simulink model "SC_RHONN"  (R2024b)
settings: Solver=FixedStepAuto  StartTime=0.0  StopTime=inf  FixedStep=1e-5  RelTol=1e-3
model workspace (MAT data in the model file):
  test = 1
libraries: instrumentseriallib x2, simulink x2, spspowerguiLib x1
settings Model: SimulationMode=accelerator  Creator=Administrator  LastModifiedBy=l'c'c
settings RTWCC: GPUComputeCapability=3.5

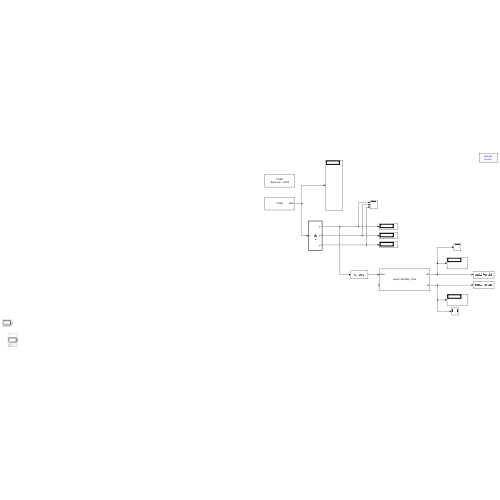
[thumbnail: Simulink's stored preview of the top-level diagram]
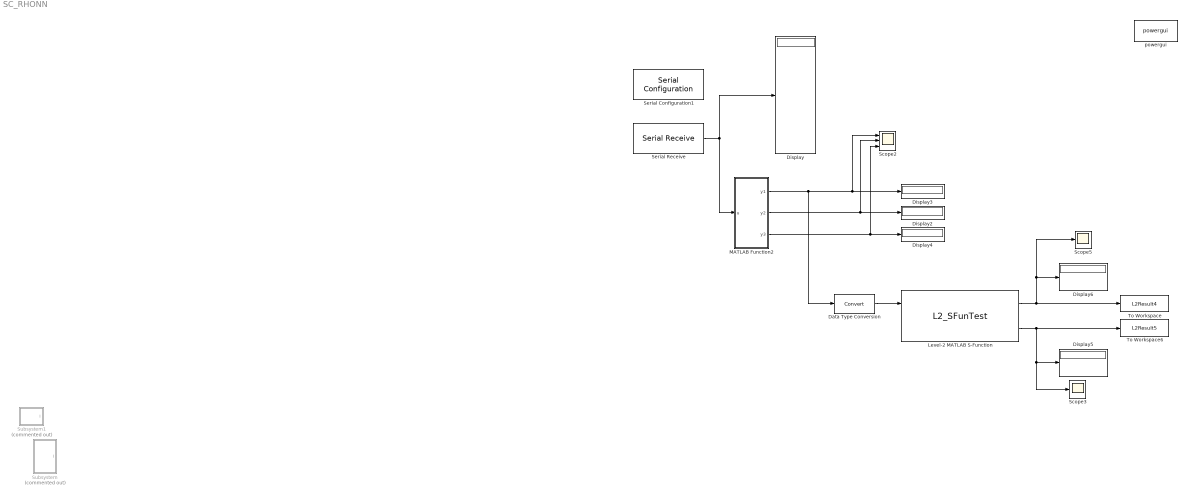
== system SC_RHONN ==
  Data Type Conversion : DataTypeConversion  SaturateOnIntegerOverflow=off  RndMeth=Floor
  Display{,2..6} (6 alike) : Display
      Display2 settings: Format=short_e
      Display3 settings: Format=short_e
      Display4 settings: Format=short_e
      Display5 settings: Priority=2
      Display6 settings: Priority=2
  Level-2 MATLAB S-Function : M-S-Function  Priority=1  FunctionName=L2_SFunTest  Parameters=Initial_Kp,Initial_Ki,Node_Num,Order_Num,Output_Num,kP_k,kQ,kR,cita  mask{Initial_Kp=0.75, Initial_Ki=20, Node_Num=2, Order_Num=3, Output_Num=2, kP_k=0.0001, kQ=0.001, kR=0.0011, cita=0.1}
      mask prompts: Initial_Kp "Initial Value of Kp"; Initial_Ki "Initial Value of Ki"; Node_Num "Node Number of RHONN"; Order_Num "Order Number of RHONN"; Output_Num "Output Number of RHONN"; kP_k "kP_k of RHONN"; kQ "kQ of RHONN"; kR "kR of RHONN"; cita "cita of RHONN"
      mask DialogControl ParameterGroupVar Prompt: 参数
      mask Display:
      | port_label('output', 1, 'Kp');
      | port_label('output', 2, 'Ki');
      | port_label('input', 1, 'Error');
      | 
      | disp('Level2_RHONN_CTRL');
  MATLAB Function2 : MATLAB Function  TreatAsAtomicUnit=on
  Scope2 : Scope  NumInputPorts=3
  Scope3 : Scope
  Scope5 : Scope
  Serial Configuration1 : instrumentseriallib/Serial Configuration  Priority=-200000  PortSel=COM5  Port=COM5  ComPort=COM5  BaudRate=19200  DataBits=8  Parity=none  StopBits=1  ByteOrder=little-endian  FlowControl=none  Timeout=1.0  SimulateUsing=Interpreted execution  BlockInModel=on  aMode=1
  Serial Receive : instrumentseriallib/Serial Receive  Priority=1  PortSel=COM5  Port=COM5  ComPort=COM5  DataType=int8  SaveDataType=uint8  ToggleHeader=off  Header=[]  ToggleDataSize=on  DataSize=[12 1]  ToggleTerminator=off  Terminator=<none>  CustomTerminator=[]  InputFormat=Column major  EnableBlockingMode=on  ActionDataUnavailable=Output last received value  ActionWhenDataUnavailable=Output last received value  CustomValue=0  SampleTime=-1  SimulateUsing=Interpreted execution  BlockInModel=on  aMode=1
  Subsystem : Subsystem  Commented=on
  Subsystem1 : Subsystem  Commented=on
  To Workspace : ToWorkspace  VariableName=L2Result4  SaveFormat=Timeseries  SampleTime=-1
  To Workspace6 : ToWorkspace  VariableName=L2Result5  SaveFormat=Timeseries  SampleTime=-1
  powergui : spspowerguiLib/powergui  Priority=1  SimulationMode=Discrete  SampleTime=1e-5  frequency=60  Iterations=50  frequencyindice=50  Pbase=100e6  ErrMax=1e-4  UnitsV=kV  UnitsW=MW  buscounter=0  FunctionMessages=off  echomessages=off  EnableUseOfTLC=off  CurrentSourceSwitches=off  DisableSnubberDevices=off  DisableRonSwitches=off  DisableVfSwitches=off  DisplayEquations=off  AutomaticDiscreteSolvers=off  SolverType=Tustin/Backward Euler (TBE)  Interpol=off  ExternalGateDelay=off  methode=off  Ts=100  x0status=blocks  SPID=on  SwTol=0  HookPort=off  NonlinearTolerance=1e-4  nMaxIteration=100  ContinueOnMaxIteration=off  RestoreLinks=warning  ResistiveCurrentMeasurement=off  Frange=[0:2:500]  Ylog=off  Xlog=on  ShowGrid=off  save=off  variable=ZData  structure=0  ZoomFFT=off  StartTime=0.0  cycles=1  DisplayStyle=1  fundamental=60  FreqAxis=off  MaxFrequency=1000  frequencyindicesteady=1  RmsSteady=1  display=off
  wires:
  Serial Receive/1 -> Display/1, MATLAB Function2/1(u)
  MATLAB Function2/3(y3) -> Scope2/3, Display4/1
  Level-2 MATLAB S-Function/1 -> Scope5/1, Display6/1, To Workspace/1
  Level-2 MATLAB S-Function/2 -> To Workspace6/1, Scope3/1, Display5/1
  Data Type Conversion/1 -> Level-2 MATLAB S-Function/1
  MATLAB Function2/1(y1) -> Scope2/1, Display3/1, Data Type Conversion/1
  MATLAB Function2/2(y2) -> Scope2/2, Display2/1

== system SC_RHONN/Subsystem ==
  Add2 : Sum  Inputs=++++
  Sine Wave3 : Sin  Amplitude=6  Frequency=2*pi*50  SampleTime=0
  Subsystem1 : Subsystem
  Subsystem6 : Subsystem
  Subsystem7 : Subsystem
  I : Outport
  wires:
  Subsystem6/1(Out1) -> Add2/4
  Subsystem1/1(Out1) -> Add2/3
  Add2/1 -> I/1
  Sine Wave3/1 -> Add2/1
  Subsystem7/1(Out1) -> Add2/2

== system SC_RHONN/Subsystem1 ==
  Add2 : Sum  Inputs=++++
  Constant : Constant  Value=400
  Subsystem1 : Subsystem
  Subsystem6 : Subsystem  Commented=on
  Subsystem7 : Subsystem
  I : Outport
  wires:
  Subsystem6/1(Out1) -> Add2/4
  Subsystem1/1(Out1) -> Add2/3
  Add2/1 -> I/1
  Constant/1 -> Add2/1
  Subsystem7/1(Out1) -> Add2/2

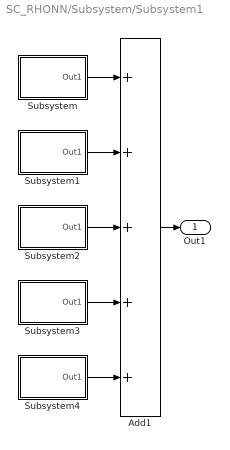
== system SC_RHONN/Subsystem/Subsystem1 ==
  Add1 : Sum  Inputs=+++++
  Subsystem : Subsystem
  Subsystem1 : Subsystem
  Subsystem2 : Subsystem
  Subsystem3 : Subsystem
  Subsystem4 : Subsystem
  Out1 : Outport
  wires:
  Subsystem1/1(Out1) -> Add1/2
  Subsystem3/1(Out1) -> Add1/4
  Subsystem4/1(Out1) -> Add1/5
  Subsystem2/1(Out1) -> Add1/3
  Subsystem/1(Out1) -> Add1/1
  Add1/1 -> Out1/1

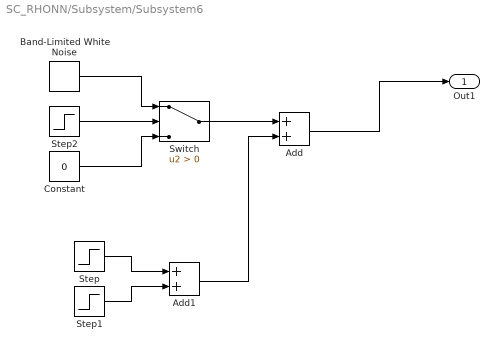
== system SC_RHONN/Subsystem/Subsystem6 ==
  Add : Sum
  Add1 : Sum
  Band-Limited White Noise : simulink/Sources/Band-Limited White Noise  Cov=[1e-5]  Ts=1e-3  seed=[23341]
  Constant : Constant  Value=0
  Step : Step  Time=0.024  After=0.3  SampleTime=0
  Step1 : Step  Time=0.026  After=-0.3  SampleTime=0
  Step2 : Step  Time=0.02  Before=1  After=0  SampleTime=0
  Switch : Switch  Criteria=u2 > Threshold  SaturateOnIntegerOverflow=off  InputSameDT=off
  Out1 : Outport
  wires:
  Add/1 -> Out1/1
  Step/1 -> Add1/1
  Constant/1 -> Switch/3
  Step1/1 -> Add1/2
  Step2/1 -> Switch/2
  Band-Limited White Noise/1 -> Switch/1
  Switch/1 -> Add/1
  Add1/1 -> Add/2

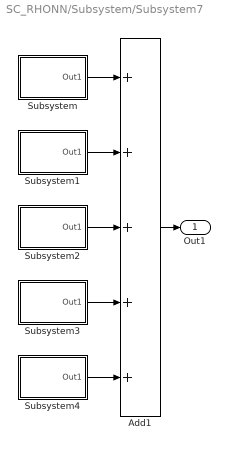
== system SC_RHONN/Subsystem/Subsystem7 ==
  Add1 : Sum  Inputs=+++++
  Subsystem : Subsystem
  Subsystem1 : Subsystem
  Subsystem2 : Subsystem
  Subsystem3 : Subsystem
  Subsystem4 : Subsystem
  Out1 : Outport
  wires:
  Add1/1 -> Out1/1
  Subsystem/1(Out1) -> Add1/1
  Subsystem2/1(Out1) -> Add1/3
  Subsystem4/1(Out1) -> Add1/5
  Subsystem3/1(Out1) -> Add1/4
  Subsystem1/1(Out1) -> Add1/2

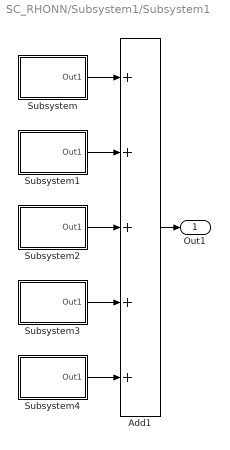
== system SC_RHONN/Subsystem1/Subsystem1 ==
  Add1 : Sum  Inputs=+++++
  Subsystem : Subsystem
  Subsystem1 : Subsystem
  Subsystem2 : Subsystem
  Subsystem3 : Subsystem
  Subsystem4 : Subsystem
  Out1 : Outport
  wires:
  Subsystem1/1(Out1) -> Add1/2
  Subsystem3/1(Out1) -> Add1/4
  Subsystem4/1(Out1) -> Add1/5
  Subsystem2/1(Out1) -> Add1/3
  Subsystem/1(Out1) -> Add1/1
  Add1/1 -> Out1/1

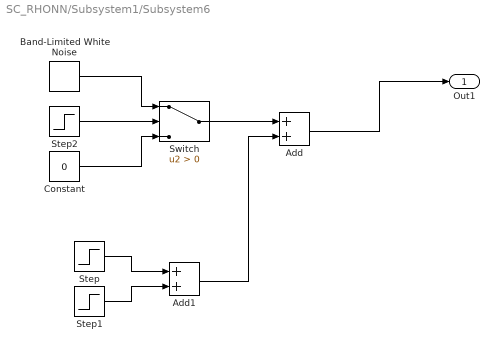
== system SC_RHONN/Subsystem1/Subsystem6 ==
  Add : Sum
  Add1 : Sum
  Band-Limited White Noise : simulink/Sources/Band-Limited White Noise  Cov=[1e-6]  Ts=0.0001  seed=[23341]
  Constant : Constant  Value=0
  Step : Step  Time=0.024  After=0.3  SampleTime=0
  Step1 : Step  Time=0.026  After=-0.3  SampleTime=0
  Step2 : Step  Time=0.02  Before=1  After=0  SampleTime=0
  Switch : Switch  Criteria=u2 > Threshold  SaturateOnIntegerOverflow=off  InputSameDT=off
  Out1 : Outport
  wires:
  Add/1 -> Out1/1
  Step/1 -> Add1/1
  Constant/1 -> Switch/3
  Step1/1 -> Add1/2
  Step2/1 -> Switch/2
  Band-Limited White Noise/1 -> Switch/1
  Switch/1 -> Add/1
  Add1/1 -> Add/2

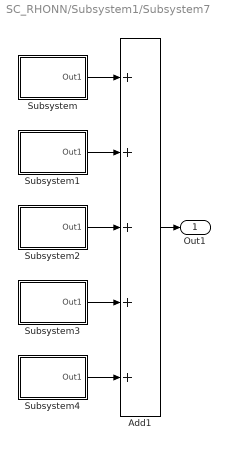
== system SC_RHONN/Subsystem1/Subsystem7 ==
  Add1 : Sum  Inputs=+++++
  Subsystem : Subsystem
  Subsystem1 : Subsystem
  Subsystem2 : Subsystem
  Subsystem3 : Subsystem
  Subsystem4 : Subsystem
  Out1 : Outport
  wires:
  Add1/1 -> Out1/1
  Subsystem/1(Out1) -> Add1/1
  Subsystem2/1(Out1) -> Add1/3
  Subsystem4/1(Out1) -> Add1/5
  Subsystem3/1(Out1) -> Add1/4
  Subsystem1/1(Out1) -> Add1/2

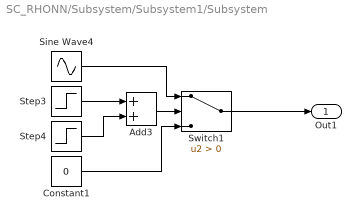
== system SC_RHONN/Subsystem/Subsystem1/Subsystem ==
  Add3 : Sum
  Constant1 : Constant  Value=0
  Sine Wave4 : Sin  Amplitude=6  Frequency=2*pi*50  Phase=pi  SampleTime=0
  Step3 : Step  Time=0.6  SampleTime=0
  Step4 : Step  Time=0.62  After=-1  SampleTime=0
  Switch1 : Switch  Criteria=u2 > Threshold  SaturateOnIntegerOverflow=off  InputSameDT=off
  Out1 : Outport
  wires:
  Switch1/1 -> Out1/1
  Step3/1 -> Add3/1
  Step4/1 -> Add3/2
  Add3/1 -> Switch1/2
  Sine Wave4/1 -> Switch1/1
  Constant1/1 -> Switch1/3

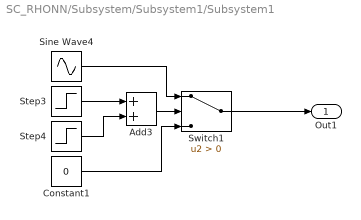
== system SC_RHONN/Subsystem/Subsystem1/Subsystem1 ==
  Add3 : Sum
  Constant1 : Constant  Value=0
  Sine Wave4 : Sin  Amplitude=5  Frequency=2*pi*50  Phase=pi  SampleTime=0
  Step3 : Step  Time=0.62  SampleTime=0
  Step4 : Step  Time=0.64  After=-1  SampleTime=0
  Switch1 : Switch  Criteria=u2 > Threshold  SaturateOnIntegerOverflow=off  InputSameDT=off
  Out1 : Outport
  wires:
  Constant1/1 -> Switch1/3
  Sine Wave4/1 -> Switch1/1
  Add3/1 -> Switch1/2
  Step4/1 -> Add3/2
  Step3/1 -> Add3/1
  Switch1/1 -> Out1/1

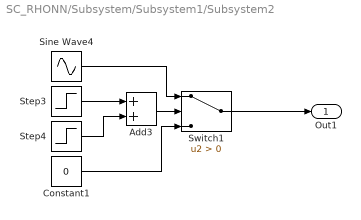
== system SC_RHONN/Subsystem/Subsystem1/Subsystem2 ==
  Add3 : Sum
  Constant1 : Constant  Value=0
  Sine Wave4 : Sin  Amplitude=4  Frequency=2*pi*50  Phase=pi  SampleTime=0
  Step3 : Step  Time=0.64  SampleTime=0
  Step4 : Step  Time=0.66  After=-1  SampleTime=0
  Switch1 : Switch  Criteria=u2 > Threshold  SaturateOnIntegerOverflow=off  InputSameDT=off
  Out1 : Outport
  wires:
  Switch1/1 -> Out1/1
  Step3/1 -> Add3/1
  Step4/1 -> Add3/2
  Add3/1 -> Switch1/2
  Sine Wave4/1 -> Switch1/1
  Constant1/1 -> Switch1/3

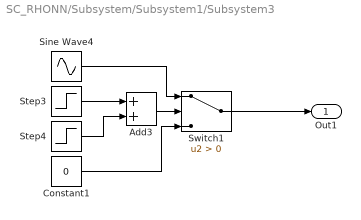
== system SC_RHONN/Subsystem/Subsystem1/Subsystem3 ==
  Add3 : Sum
  Constant1 : Constant  Value=0
  Sine Wave4 : Sin  Amplitude=3  Frequency=2*pi*50  Phase=pi  SampleTime=0
  Step3 : Step  Time=0.66  SampleTime=0
  Step4 : Step  Time=0.68  After=-1  SampleTime=0
  Switch1 : Switch  Criteria=u2 > Threshold  SaturateOnIntegerOverflow=off  InputSameDT=off
  Out1 : Outport
  wires:
  Constant1/1 -> Switch1/3
  Sine Wave4/1 -> Switch1/1
  Add3/1 -> Switch1/2
  Step4/1 -> Add3/2
  Step3/1 -> Add3/1
  Switch1/1 -> Out1/1

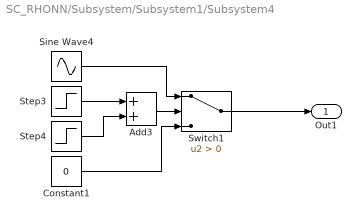
== system SC_RHONN/Subsystem/Subsystem1/Subsystem4 ==
  Add3 : Sum
  Constant1 : Constant  Value=0
  Sine Wave4 : Sin  Amplitude=2  Frequency=2*pi*50  Phase=pi  SampleTime=0
  Step3 : Step  Time=0.68  SampleTime=0
  Step4 : Step  Time=0.7  After=-1  SampleTime=0
  Switch1 : Switch  Criteria=u2 > Threshold  SaturateOnIntegerOverflow=off  InputSameDT=off
  Out1 : Outport
  wires:
  Switch1/1 -> Out1/1
  Step3/1 -> Add3/1
  Step4/1 -> Add3/2
  Add3/1 -> Switch1/2
  Sine Wave4/1 -> Switch1/1
  Constant1/1 -> Switch1/3

== system SC_RHONN/Subsystem/Subsystem7/Subsystem ==
  Add3 : Sum
  Constant1 : Constant  Value=0
  Sine Wave4 : Sin  Amplitude=6  Frequency=2*pi*50  Phase=2*pi  SampleTime=0
  Step3 : Step  Time=0.2  SampleTime=0
  Step4 : Step  Time=0.22  After=-1  SampleTime=0
  Switch1 : Switch  Criteria=u2 > Threshold  SaturateOnIntegerOverflow=off  InputSameDT=off
  Out1 : Outport
  wires:
  Constant1/1 -> Switch1/3
  Sine Wave4/1 -> Switch1/1
  Add3/1 -> Switch1/2
  Step4/1 -> Add3/2
  Step3/1 -> Add3/1
  Switch1/1 -> Out1/1

== system SC_RHONN/Subsystem/Subsystem7/Subsystem1 ==
  Add3 : Sum
  Constant1 : Constant  Value=0
  Sine Wave4 : Sin  Amplitude=5  Frequency=2*pi*50  Phase=2*pi  SampleTime=0
  Step3 : Step  Time=0.22  SampleTime=0
  Step4 : Step  Time=0.24  After=-1  SampleTime=0
  Switch1 : Switch  Criteria=u2 > Threshold  SaturateOnIntegerOverflow=off  InputSameDT=off
  Out1 : Outport
  wires:
  Switch1/1 -> Out1/1
  Step3/1 -> Add3/1
  Step4/1 -> Add3/2
  Add3/1 -> Switch1/2
  Sine Wave4/1 -> Switch1/1
  Constant1/1 -> Switch1/3

== system SC_RHONN/Subsystem/Subsystem7/Subsystem2 ==
  Add3 : Sum
  Constant1 : Constant  Value=0
  Sine Wave4 : Sin  Amplitude=4  Frequency=2*pi*50  Phase=2*pi  SampleTime=0
  Step3 : Step  Time=0.24  SampleTime=0
  Step4 : Step  Time=0.26  After=-1  SampleTime=0
  Switch1 : Switch  Criteria=u2 > Threshold  SaturateOnIntegerOverflow=off  InputSameDT=off
  Out1 : Outport
  wires:
  Constant1/1 -> Switch1/3
  Sine Wave4/1 -> Switch1/1
  Add3/1 -> Switch1/2
  Step4/1 -> Add3/2
  Step3/1 -> Add3/1
  Switch1/1 -> Out1/1

== system SC_RHONN/Subsystem/Subsystem7/Subsystem3 ==
  Add3 : Sum
  Constant1 : Constant  Value=0
  Sine Wave4 : Sin  Amplitude=3  Frequency=2*pi*50  Phase=2*pi  SampleTime=0
  Step3 : Step  Time=0.26  SampleTime=0
  Step4 : Step  Time=0.28  After=-1  SampleTime=0
  Switch1 : Switch  Criteria=u2 > Threshold  SaturateOnIntegerOverflow=off  InputSameDT=off
  Out1 : Outport
  wires:
  Switch1/1 -> Out1/1
  Step3/1 -> Add3/1
  Step4/1 -> Add3/2
  Add3/1 -> Switch1/2
  Sine Wave4/1 -> Switch1/1
  Constant1/1 -> Switch1/3

== system SC_RHONN/Subsystem/Subsystem7/Subsystem4 ==
  Add3 : Sum
  Constant1 : Constant  Value=0
  Sine Wave4 : Sin  Amplitude=2  Frequency=2*pi*50  Phase=2*pi  SampleTime=0
  Step3 : Step  Time=0.28  SampleTime=0
  Step4 : Step  Time=0.3  After=-1  SampleTime=0
  Switch1 : Switch  Criteria=u2 > Threshold  SaturateOnIntegerOverflow=off  InputSameDT=off
  Out1 : Outport
  wires:
  Constant1/1 -> Switch1/3
  Sine Wave4/1 -> Switch1/1
  Add3/1 -> Switch1/2
  Step4/1 -> Add3/2
  Step3/1 -> Add3/1
  Switch1/1 -> Out1/1

== system SC_RHONN/Subsystem1/Subsystem1/Subsystem ==
  Add3 : Sum
  Constant1 : Constant  Value=0
  Constant2 : Constant  Value=-10
  Step3 : Step  Time=0.6  SampleTime=0
  Step4 : Step  Time=0.62  After=-1  SampleTime=0
  Switch1 : Switch  Criteria=u2 > Threshold  SaturateOnIntegerOverflow=off  InputSameDT=off
  Out1 : Outport
  wires:
  Switch1/1 -> Out1/1
  Step3/1 -> Add3/1
  Step4/1 -> Add3/2
  Add3/1 -> Switch1/2
  Constant2/1 -> Switch1/1
  Constant1/1 -> Switch1/3

== system SC_RHONN/Subsystem1/Subsystem1/Subsystem1 ==
  Add3 : Sum
  Constant1 : Constant  Value=0
  Constant2 : Constant  Value=-8
  Step3 : Step  Time=0.62  SampleTime=0
  Step4 : Step  Time=0.64  After=-1  SampleTime=0
  Switch1 : Switch  Criteria=u2 > Threshold  SaturateOnIntegerOverflow=off  InputSameDT=off
  Out1 : Outport
  wires:
  Constant1/1 -> Switch1/3
  Constant2/1 -> Switch1/1
  Add3/1 -> Switch1/2
  Step4/1 -> Add3/2
  Step3/1 -> Add3/1
  Switch1/1 -> Out1/1

== system SC_RHONN/Subsystem1/Subsystem1/Subsystem2 ==
  Add3 : Sum
  Constant1 : Constant  Value=0
  Constant2 : Constant  Value=-6
  Step3 : Step  Time=0.64  SampleTime=0
  Step4 : Step  Time=0.66  After=-1  SampleTime=0
  Switch1 : Switch  Criteria=u2 > Threshold  SaturateOnIntegerOverflow=off  InputSameDT=off
  Out1 : Outport
  wires:
  Switch1/1 -> Out1/1
  Step3/1 -> Add3/1
  Step4/1 -> Add3/2
  Add3/1 -> Switch1/2
  Constant2/1 -> Switch1/1
  Constant1/1 -> Switch1/3

== system SC_RHONN/Subsystem1/Subsystem1/Subsystem3 ==
  Add3 : Sum
  Constant1 : Constant  Value=0
  Constant2 : Constant  Value=-4
  Step3 : Step  Time=0.66  SampleTime=0
  Step4 : Step  Time=0.68  After=-1  SampleTime=0
  Switch1 : Switch  Criteria=u2 > Threshold  SaturateOnIntegerOverflow=off  InputSameDT=off
  Out1 : Outport
  wires:
  Constant1/1 -> Switch1/3
  Add3/1 -> Switch1/2
  Step4/1 -> Add3/2
  Step3/1 -> Add3/1
  Switch1/1 -> Out1/1
  Constant2/1 -> Switch1/1

== system SC_RHONN/Subsystem1/Subsystem1/Subsystem4 ==
  Add3 : Sum
  Constant1 : Constant  Value=0
  Constant2 : Constant  Value=-2
  Step3 : Step  Time=0.68  SampleTime=0
  Step4 : Step  Time=0.7  After=-1  SampleTime=0
  Switch1 : Switch  Criteria=u2 > Threshold  SaturateOnIntegerOverflow=off  InputSameDT=off
  Out1 : Outport
  wires:
  Switch1/1 -> Out1/1
  Step3/1 -> Add3/1
  Step4/1 -> Add3/2
  Add3/1 -> Switch1/2
  Constant2/1 -> Switch1/1
  Constant1/1 -> Switch1/3

== system SC_RHONN/Subsystem1/Subsystem7/Subsystem ==
  Add3 : Sum
  Constant : Constant  Value=10
  Constant1 : Constant  Value=0
  Step3 : Step  Time=0  SampleTime=0
  Step4 : Step  Time=0.22  After=-1  SampleTime=0
  Switch1 : Switch  Criteria=u2 > Threshold  SaturateOnIntegerOverflow=off  InputSameDT=off
  Out1 : Outport
  wires:
  Constant1/1 -> Switch1/3
  Constant/1 -> Switch1/1
  Add3/1 -> Switch1/2
  Step4/1 -> Add3/2
  Step3/1 -> Add3/1
  Switch1/1 -> Out1/1

== system SC_RHONN/Subsystem1/Subsystem7/Subsystem1 ==
  Add3 : Sum
  Constant : Constant  Value=8
  Constant1 : Constant  Value=0
  Step3 : Step  Time=0.22  SampleTime=0
  Step4 : Step  Time=0.24  After=-1  SampleTime=0
  Switch1 : Switch  Criteria=u2 > Threshold  SaturateOnIntegerOverflow=off  InputSameDT=off
  Out1 : Outport
  wires:
  Switch1/1 -> Out1/1
  Step3/1 -> Add3/1
  Step4/1 -> Add3/2
  Add3/1 -> Switch1/2
  Constant/1 -> Switch1/1
  Constant1/1 -> Switch1/3

== system SC_RHONN/Subsystem1/Subsystem7/Subsystem2 ==
  Add3 : Sum
  Constant : Constant  Value=6
  Constant1 : Constant  Value=0
  Step3 : Step  Time=0.24  SampleTime=0
  Step4 : Step  Time=0.26  After=-1  SampleTime=0
  Switch1 : Switch  Criteria=u2 > Threshold  SaturateOnIntegerOverflow=off  InputSameDT=off
  Out1 : Outport
  wires:
  Constant1/1 -> Switch1/3
  Constant/1 -> Switch1/1
  Add3/1 -> Switch1/2
  Step4/1 -> Add3/2
  Step3/1 -> Add3/1
  Switch1/1 -> Out1/1

== system SC_RHONN/Subsystem1/Subsystem7/Subsystem3 ==
  Add3 : Sum
  Constant : Constant  Value=4
  Constant1 : Constant  Value=0
  Step3 : Step  Time=0.26  SampleTime=0
  Step4 : Step  Time=0.28  After=-1  SampleTime=0
  Switch1 : Switch  Criteria=u2 > Threshold  SaturateOnIntegerOverflow=off  InputSameDT=off
  Out1 : Outport
  wires:
  Switch1/1 -> Out1/1
  Step3/1 -> Add3/1
  Step4/1 -> Add3/2
  Add3/1 -> Switch1/2
  Constant/1 -> Switch1/1
  Constant1/1 -> Switch1/3

== system SC_RHONN/Subsystem1/Subsystem7/Subsystem4 ==
  Add3 : Sum
  Constant : Constant  Value=2
  Constant1 : Constant  Value=0
  Step3 : Step  Time=0.28  SampleTime=0
  Step4 : Step  Time=0.3  After=-1  SampleTime=0
  Switch1 : Switch  Criteria=u2 > Threshold  SaturateOnIntegerOverflow=off  InputSameDT=off
  Out1 : Outport
  wires:
  Constant1/1 -> Switch1/3
  Add3/1 -> Switch1/2
  Step4/1 -> Add3/2
  Step3/1 -> Add3/1
  Switch1/1 -> Out1/1
  Constant/1 -> Switch1/1

== matlab function SC_RHONN/MATLAB Function2 ==
  data: u input; y1 output; y2 output; y3 output
function [y1,y2,y3] = fcn(u)
u1 = single(u);
y1 = u1(1)+(u1(2))/10.0+(u1(3))/100.0+(u1(4))/1000.0;
y2 = (u1(5))+(u1(6))/10.0+(u1(7))/100.0+(u1(8))/1000.0;
y3 = (u1(9))+(u1(10))/10.0+(u1(11))/100.0+(u1(12))/1000.0;
end
